simulink model "HSat_orbit_merged_maria"  (R2023b)
settings: Solver=FixedStepAuto  StartTime=0  StopTime=86400*900  MaxStep=3600  RelTol=1e-3  EnableMultiTasking=on
values from neighbouring files (symbols this model uses):
  alpha_acc = sqrt(0.7)    [HSat_op_setup_merged_maria.m]    (also in init_orbit_analysis_with_drag_loss.m)
  ext_ENV_G = 6.674e-11    [HSat_op_setup.m]    (also in HSat_op_setup_merged_maria.m)
  ext_ENV_muEarth = 3.986005e14    (= 398600500000000)    [GEO_insertion_setup.m]    (also in HSat_op_setup.m; HSat_op_setup_merged_maria.m; init_orbit_analysis_with_drag_loss.m)
  ext_ENV_Re = 6.37813700*10^6    (= 6378137)    [HSat_op_setup.m]    (also in HSat_op_setup_merged_maria.m)
  ext_EOR_atmosphere_end = 1000e3    (= 1000000)    [HSat_op_setup.m]    (also in HSat_op_setup_merged_maria.m)
  ext_EOR_perigeeraise_end = 600e3    (= 600000)    [HSat_op_setup.m]    (also in HSat_op_setup_merged_maria.m)
  ext_Main_initDate_IC_T = sim_start    [HSat_op_setup.m]    (also in HSat_op_setup_merged_maria.m)
  ext_SC_activecorr_COE_ECI = [1, 1, 1, 0, 0, 0, 0, 0 ]    [HSat_op_setup.m]    (also in HSat_op_setup_merged_maria.m)
  ext_SC_balanced_COE_ECI = [ .500    0.70    1.100 1 1]    [HSat_op_setup.m]    (also in HSat_op_setup_merged_maria.m = [ 0.10 2.10 1.40    1.0000    1.0000]; launch_settings.m)
  ext_SC_cutofferror_COE_ECI = [150e3, .01, 0.1*pi/180, .1*pi/180,.1*pi/180, 0, 0, 0]    [HSat_op_setup.m]    (also in HSat_op_setup_merged_maria.m)
  ext_SC_init_COE_ECI = [a0,ecc0,i0,an0,ap0,tran0,eccan0,ma0]    [HSat_op_setup.m]    (also in HSat_op_setup_merged_maria.m)
  ext_SC_target_COE_ECI = [a1,ecc1,i1,an1,ap1,tran1,eccan1,ma1]    [HSat_op_setup.m]    (also in HSat_op_setup_merged_maria.m)
  ext_SC_target_lambda = 67*pi/180    (= 1.16937059884)    [HSat_op_setup.m]    (also in HSat_op_setup_merged_maria.m)
  flip_timer = 2*60*60    (= 7200)    [HSat_op_setup_merged_maria.m]
  P_solar = 4.56e-6    (= 4.56e-06)    [HSat_op_setup_merged_maria.m]    (also in init_orbit_analysis_with_drag_loss.m)
  sim_SC_init_CoG_EOR_dry = [-0.00448 0.00106 0.46931]    [HSat_op_setup.m]    (also in HSat_op_setup_merged_maria.m)
  sim_SC_init_CoG_propellant = [0 0 0.24758]    [HSat_op_setup.m]    (also in HSat_op_setup_merged_maria.m)
  sim_SC_init_dry_mass = sim_SC_init_wet_mass-sim_SC_init_propellant_mass    (= 727)    [HSat_op_setup.m]    (also in HSat_op_setup_merged_maria.m = 813.7)
  sim_SC_init_MoI_EOR_wet = [ ... (first row only)    [HSat_op_setup.m]    (also in HSat_op_setup_merged_maria.m; init_orbit_analysis_with_drag_loss.m)
  sim_SC_init_wet_mass = 750    [HSat_op_setup.m]    (also in HSat_op_setup_merged_maria.m)
  sim_thrust_force = [ ... (first row only)    [HSat_op_setup.m]    (also in HSat_op_setup_merged_maria.m)
  sim_thrust_massflow = [ ... (first row only)    [HSat_op_setup.m]    (also in HSat_op_setup_merged_maria.m)
  sim_thrust_vector = [ ... (first row only)    [HSat_op_setup.m]    (also in HSat_op_setup_merged_maria.m)
  sim_thruster_position = [ ... (first row only)    [HSat_op_setup.m]    (also in HSat_op_setup_merged_maria.m)
  sim_ts_save = 60    [HSat_op_setup.m]    (also in HSat_op_setup_merged_maria.m)
  sun_pointing_SA = 0    [HSat_op_setup_merged_maria.m]    (also in init_orbit_analysis_with_drag_loss.m)
  third_body_jupiter = 1    [HSat_op_setup.m]    (also in HSat_op_setup_merged_maria.m)
  third_body_moon = 1    [HSat_op_setup.m]    (also in HSat_op_setup_merged_maria.m)
  third_body_sun = 1    [HSat_op_setup.m]    (also in HSat_op_setup_merged_maria.m)
libraries: aerolibutil x59, simulink x18, matrix_library x16, Toolbox x10, sharedtransform x9, sharedutil x5, aerolibatmos2 x1, simulink_extras x1
(part 2 of 8)

== system HSat_orbit_merged_maria/Subsystem1/Navigation/q_slo ==
  posECI : Inport
  velECI : Inport  Port=2
  Create 3x3 Matrix : sharedutil/Create 3x3 Matrix  aMode=aMode
      settings: LibrarySourceBlock=aerolibutil/Create 3x3 Matrix
  Demux : Demux  Outputs=3
  Demux1 : Demux  Outputs=3
  Demux2 : Demux  Outputs=3
  Direction Cosine Matrix to Quaternions : sharedtransform/Direction Cosine Matrix  to Quaternions  aMode=0  action=None  tolerance=eps(2)
      settings: LibrarySourceBlock=|
      | aerolibtransform2/Direction Cosine Matrix
      | to Quaternions
  Unary Minus : UnaryMinus
  VecNormalize : Subsystem
      mask Display: disp('u/||u||')
  VecNormalize1 : Subsystem
      mask Display: disp('u/||u||')
  VecNormalize2 : Subsystem
      mask Display: disp('u/||u||')
  VecNormalize3 : Subsystem
      mask Display: disp('u/||u||')
  Z x R : Subsystem  mask(Cross Product){}
      mask help: Calculates the cross product of two 3x1 vectors.
      mask Help:
      | <p>This block calculates the cross product of two 3x1 vectors, ie.</p>
      | 
      | <ul>C(1) = A(2)*B(3) - A(3)*B(2)</ul>
      | <ul>C(2) = A(3)*B(1) - A(1)*B(3)</ul>
      | <ul>C(3) = A(1)*B(2) - A(2)*B(1)</ul>
      | 
      | <p>The block inputs and output contain more than one signal as described below.</p>
      | 
      | <p><H4>Block Vector Input 1 - A</H4>
      | <ul>
      | <li>A(1)</li>
      | <li>A(2)</li>
      | <li>A(3)</li>
      | </ul>
      | </p>
      | 
      | <p><H4>Block Vector Input 2 - B</H4>
      | <ul>
      | <li>B(1)</li>
      | <li>B(2)</li>
      | <li>B(3)</li>
      | </ul>
      | </p>
      | 
      | <p><H4>Block Vector Output - Cross Product (AxB)</H4>
      | <ul>
      | <li>C(1)</li>
      | <li>C(2)</li>
      | <li>C(3)</li>
      | </ul>
      | </p>
      mask Display: disp('Cross\nProduct')
  Z x Y : Subsystem  mask(Cross Product){}
      mask help: Calculates the cross product of two 3x1 vectors.
      mask Help:
      | <p>This block calculates the cross product of two 3x1 vectors, ie.</p>
      | 
      | <ul>C(1) = A(2)*B(3) - A(3)*B(2)</ul>
      | <ul>C(2) = A(3)*B(1) - A(1)*B(3)</ul>
      | <ul>C(3) = A(1)*B(2) - A(2)*B(1)</ul>
      | 
      | <p>The block inputs and output contain more than one signal as described below.</p>
      | 
      | <p><H4>Block Vector Input 1 - A</H4>
      | <ul>
      | <li>A(1)</li>
      | <li>A(2)</li>
      | <li>A(3)</li>
      | </ul>
      | </p>
      | 
      | <p><H4>Block Vector Input 2 - B</H4>
      | <ul>
      | <li>B(1)</li>
      | <li>B(2)</li>
      | <li>B(3)</li>
      | </ul>
      | </p>
      | 
      | <p><H4>Block Vector Output - Cross Product (AxB)</H4>
      | <ul>
      | <li>C(1)</li>
      | <li>C(2)</li>
      | <li>C(3)</li>
      | </ul>
      | </p>
      mask Display: disp('Cross\nProduct')
  qECI2slo : Outport  InitialOutput=0
  wires:
  Unary Minus/1 -> Z x Y/2(b(1) b(2) b(3)), Demux2/1, Z x R/1(a(1) a(2) a(3))  "Z"
  posECI/1 -> VecNormalize3/1(In1)
  VecNormalize3/1(Out1) -> Unary Minus/1
  velECI/1 -> VecNormalize2/1(In1)
  VecNormalize2/1(Out1) -> Z x R/2(b(1) b(2) b(3))
  Z x R/1(c(1) c(2) c(3)) -> VecNormalize1/1(In1)
  VecNormalize1/1(Out1) -> Z x Y/1(a(1) a(2) a(3)), Demux1/1  "Y"
  Z x Y/1(c(1) c(2) c(3)) -> VecNormalize/1(In1)
  VecNormalize/1(Out1) -> Demux/1  "X"
  Demux/1 -> Create 3x3 Matrix/1
  Demux/2 -> Create 3x3 Matrix/2
  Demux/3 -> Create 3x3 Matrix/3
  Demux1/1 -> Create 3x3 Matrix/4
  Demux1/2 -> Create 3x3 Matrix/5
  Demux1/3 -> Create 3x3 Matrix/6
  Demux2/1 -> Create 3x3 Matrix/7
  Demux2/2 -> Create 3x3 Matrix/8
  Demux2/3 -> Create 3x3 Matrix/9
  Create 3x3 Matrix/1 -> Direction Cosine Matrix to Quaternions/1
  Direction Cosine Matrix to Quaternions/1 -> qECI2slo/1

== system HSat_orbit_merged_maria/Subsystem1/control/EORattitude ==
  note: Not used
  AllThrustsSCB : Inport
  AmomECI : Inport  Port=2
  thrust_slo : Inport  Port=3
  sunv_eci : Inport  Port=4
  q_eci2slo : Inport  Port=5
  AllTorquesSCB1 : Inport  Port=6
  q_eci2scb : Inport  Port=7
  Bus Creator : BusCreator  Inputs=3
  Bus Creator1 : BusCreator  Inputs=3
  Bus Selector : BusSelector  OutputSignals=signal1,signal2,signal3
  Delay : Delay  DelayLength=1  InitialCondition=0
  Logical Operator : Logic  Operator=OR  AllPortsSameDT=off  OutDataTypeStr=boolean
  Logical Operator1 : Logic  Operator=NOT  AllPortsSameDT=off  OutDataTypeStr=boolean
  Logical Operator2 : Logic  AllPortsSameDT=off  OutDataTypeStr=boolean
  Manual Switch1 : ManualSwitch  CurrentSetting=0
  OR or SK unloading : Subsystem
  Subsystem : Subsystem
  Subsystem2 : Subsystem
  Subsystem4 : Subsystem
  Terminator : Terminator
  Unit Delay : UnitDelay  SampleTime=-1  HasFrameUpgradeWarning=on
  ActiveThrusters : Outport
  qECI2scb : Outport  Port=2
  DoAMOM : Outport  Port=3
  flip_unload : Outport  Port=4
  wires:
  sunv_eci/1 -> Subsystem/7(sunv_eci), Subsystem4/6(sunv_eci)
  Subsystem2/3(EORTorqueSCB) -> Subsystem4/3(EORtorqueSCB), Subsystem/4(EORtorqueSCB)
  AmomECI/1 -> OR or SK unloading/1(AmomECI), Subsystem4/1(AmomECI), Subsystem/1(AmomECI)
  Subsystem4/1(qECI2scb) -> Bus Creator1/1
  Subsystem2/2(EORForceSCB) -> Subsystem4/2(EORthrustSCB), Subsystem/3(EORthrustSCB)
  thrust_slo/1 -> Subsystem4/4(thrust_slo), Subsystem/5(thrust_slo)
  q_eci2slo/1 -> Subsystem4/5(q_eci2slo), Subsystem/6(q_slo2eci)
  Subsystem/1(qECI2scb) -> Bus Creator/1
  OR or SK unloading/1(PPU1active) -> Subsystem2/1(PPU1active)
  AllThrustsSCB/1 -> Subsystem2/2(AllThrustsSCB)
  OR or SK unloading/2(PPU2active) -> Subsystem2/3(PPU2active)
  AllTorquesSCB1/1 -> Subsystem2/4(AllTorquesSCB1)
  Subsystem2/1(ActiveThrusters) -> ActiveThrusters/1
  q_eci2scb/1 -> Subsystem/2(q_eci2scb)
  Subsystem4/2(DoAMOM) -> Bus Creator1/2
  Subsystem/2(DoAMOM) -> Bus Creator/2
  Bus Creator1/1 -> Manual Switch1/2
  Bus Creator/1 -> Manual Switch1/1
  Manual Switch1/1 -> Bus Selector/1
  Bus Selector/1 -> qECI2scb/1  "<signal1>"
  Bus Selector/2 -> Logical Operator/1  "<signal2>"
  Subsystem4/3(NoAMOM) -> Bus Creator1/3
  Subsystem/3(NoAMOM) -> Bus Creator/3
  Bus Selector/3 -> Logical Operator1/1  "<signal3>"
  Logical Operator1/1 -> Logical Operator2/2
  Logical Operator2/1 -> DoAMOM/1, Delay/1
  Delay/1 -> Logical Operator/2
  Logical Operator/1 -> Logical Operator2/1
  OR or SK unloading/3(PPUSKactive) -> Subsystem4/7(unloading_ongoing), Subsystem2/5(PPUSKactive)
  Subsystem2/4(SKThrustersActive) -> Terminator/1
  Subsystem4/5(SKunload) -> Unit Delay/1
  Unit Delay/1 -> OR or SK unloading/2(SKunload)
  Subsystem4/4(flip_unloading) -> flip_unload/1

== system HSat_orbit_merged_maria/Subsystem1/control/Subsystem6 ==
  q_eci2scb_wanted : Inport
  AllTorquesSCB : Inport  Port=2
  sunv : Inport  Port=3
  WantedTorqueECI : Inport  Port=4
  PPU1active : Inport  Port=5
  PPU2active : Inport  Port=6
  Subsystem2 : Subsystem
  active_thrusters : Outport
  q_eci2scb : Outport  Port=2
  wires:
  AllTorquesSCB/1 -> Subsystem2/3(AllTorquesSCB)
  q_eci2scb_wanted/1 -> Subsystem2/4(q_eci2scb_wanted)
  PPU1active/1 -> Subsystem2/1(PPU1active)
  PPU2active/1 -> Subsystem2/2(PPU2active)
  WantedTorqueECI/1 -> Subsystem2/5(WantedTorqueECI)
  Subsystem2/1(ActiveThrusters) -> active_thrusters/1
  Subsystem2/2(q_eci2scb) -> q_eci2scb/1
  sunv/1 -> Subsystem2/6(sunv)

== system HSat_orbit_merged_maria/Subsystem1/control/TorquesAndForces ==
  Active_thruster : Inport
  thrusting : Inport  Port=2
  SC_mass : Inport  Port=3
  Constant : Constant  Value=sim_thruster_position
  Constant1 : Constant  Value=sim_thrust_vector
  Constant2 : Constant  Value=sim_thrust_force
  Constant3 : Constant  Value=[1 1 1]
  Constant4 : Constant  Value=[1 1 1 1 1 1 1 1 1 1 1]'
  Constant5 : Constant  Value=sim_thrust_massflow
  Constant6 : Constant  Value=[1 1 1]
  Display : Display
  MATLAB Function : MATLAB Function  TreatAsAtomicUnit=on
  Product{,2,4..5,7} (5 alike) : Product
  Product1 : Product  Multiplication=Matrix(*)
  Product3 : Product  Multiplication=Matrix(*)
  Product6 : Product  Multiplication=Matrix(*)
  Reshape : Reshape  OutputDimensionality=Column vector (2-D)
  Reshape1 : Reshape  OutputDimensionality=Column vector (2-D)
  Reshape2 : Reshape  OutputDimensionality=Row vector (2-D)
  Reshape3 : Reshape  OutputDimensionality=Row vector (2-D)
  Reshape4 : Reshape  OutputDimensionality=Column vector (2-D)
  Subsystem : Subsystem
  Sum : Sum  Inputs=+-|
  Sum of Elements1 : Sum  Inputs=+  CollapseMode=Specified dimension
  Sum of Elements2 : Sum  Inputs=+  CollapseMode=Specified dimension
  Sum of Elements6 : Sum  Inputs=+  CollapseMode=Specified dimension
  EPtorqueSCB : Outport
  EPThrustSCB : Outport  Port=2
  TotalMassFlow : Outport  Port=3
  AllThrustsSCB : Outport  Port=4
  AllTorquesSCB : Outport  Port=5
  wires:
  Sum of Elements6/1 -> EPtorqueSCB/1
  Sum of Elements1/1 -> EPThrustSCB/1
  Product5/1 -> Sum of Elements6/1
  SC_mass/1 -> Subsystem/1(SC_mass)
  Constant2/1 -> Reshape1/1
  Sum/1 -> MATLAB Function/1(v)
  Subsystem/1(SC_CoG) -> Product3/2
  Reshape1/1 -> Product1/1
  Constant1/1 -> Product2/1
  Product1/1 -> Product2/2
  Constant/1 -> Sum/1
  Constant4/1 -> Product3/1
  Constant3/1 -> Reshape2/1
  Reshape2/1 -> Product1/2
  Product3/1 -> Sum/2
  Reshape4/1 -> Product4/1
  Constant5/1 -> Reshape4/1
  Product4/1 -> Sum of Elements2/1
  Sum of Elements2/1 -> TotalMassFlow/1
  Product/1 -> Sum of Elements1/1
  MATLAB Function/1(u) -> AllTorquesSCB/1, Product5/1
  Product6/1 -> Product5/2, Product/2
  Constant6/1 -> Reshape3/1
  Reshape3/1 -> Product6/2
  Reshape/1 -> Product4/2, Product6/1
  thrusting/1 -> Product7/2
  Product7/1 -> Reshape/1
  Product2/1 -> Product/1, AllThrustsSCB/1, MATLAB Function/2(w)
  Active_thruster/1 -> Display/1, Product7/1

== system HSat_orbit_merged_maria/Subsystem1/Dynamics/Subsystem/3 body perturbation legendre polynomial ==
  r_sat : Inport
  r_sun : Inport  Port=2
  r_moon : Inport  Port=3
  r_jupiter : Inport  Port=4
  Constant1 : Constant  Value=[0,0,0]
  Constant2 : Constant  Value=[0,0,0]
  Constant3 : Constant  Value=third_body_sun
  Constant4 : Constant  Value=third_body_moon
  Constant5 : Constant  Value=[0,0,0]
  Constant6 : Constant  Value=third_body_jupiter
  Legendre degree : Constant  Value=2
  Subsystem1 : Subsystem
  Subsystem2 : Subsystem
  Subsystem3 : Subsystem
  Subtract : Sum  Inputs=---
  Switch1 : Switch  Criteria=u2 > Threshold  SaturateOnIntegerOverflow=off  InputSameDT=off
  Switch2 : Switch  Criteria=u2 > Threshold  SaturateOnIntegerOverflow=off  InputSameDT=off
  Switch3 : Switch  Criteria=u2 > Threshold  SaturateOnIntegerOverflow=off  InputSameDT=off
  jupiter mass : Constant  Value=1.898e27
  moon mass : Constant  Value=7.342e22
  sun mass : Constant  Value=1.989e30
  3rdbodyacc : Outport
  wires:
  r_sat/1 -> Subsystem1/1(sat), Subsystem3/1(sat), Subsystem2/1(sat)
  r_sun/1 -> Subsystem2/2(3 body)
  sun mass/1 -> Subsystem2/3(mass)
  r_moon/1 -> Subsystem1/2(3 body)
  moon mass/1 -> Subsystem1/3(mass)
  r_jupiter/1 -> Subsystem3/2(3 body)
  jupiter mass/1 -> Subsystem3/3(mass)
  Subtract/1 -> 3rdbodyacc/1
  Legendre degree/1 -> Subsystem1/4(Legendre deg), Subsystem3/4(Legendre deg), Subsystem2/4(Legendre deg)
  Subsystem2/1(Out1) -> Switch1/1
  Switch1/1 -> Subtract/1
  Constant2/1 -> Switch1/3
  Constant3/1 -> Switch1/2
  Constant1/1 -> Switch2/3
  Switch2/1 -> Subtract/2
  Constant4/1 -> Switch2/2
  Subsystem1/1(Out1) -> Switch2/1
  Constant5/1 -> Switch3/3
  Switch3/1 -> Subtract/3
  Constant6/1 -> Switch3/2
  Subsystem3/1(Out1) -> Switch3/1

== system HSat_orbit_merged_maria/Subsystem1/Dynamics/Subsystem/Ephemeris ==
  T JD : Inport
  Gain{,1..3} (4 alike) : Gain  Gain=1000
  Jupiter Ephemeris : PlanetaryEphem  target=Jupiter
  Lunar Ephemeris : PlanetaryEphem
  Solar Ephemeris : PlanetaryEphem  target=Sun
  Terminator : Terminator
  Terminator1 : Terminator
  Terminator2 : Terminator
  km to m : Gain  Gain=1000
  km to m1 : Gain  Gain=1000
  solar_X : Outport
  lunar_X : Outport  Port=2
  jupiter_X : Outport  Port=3
  wires:
  T JD/1 -> Lunar Ephemeris/1, Jupiter Ephemeris/1, Solar Ephemeris/1
  Lunar Ephemeris/2 -> Gain1/1
  Solar Ephemeris/1 -> Gain2/1
  Solar Ephemeris/2 -> km to m/1
  Lunar Ephemeris/1 -> Gain/1
  Gain/1 -> lunar_X/1
  Gain1/1 -> Terminator2/1
  Gain2/1 -> solar_X/1
  km to m/1 -> Terminator1/1
  Jupiter Ephemeris/2 -> km to m1/1
  Gain3/1 -> jupiter_X/1
  km to m1/1 -> Terminator/1
  Jupiter Ephemeris/1 -> Gain3/1

== system HSat_orbit_merged_maria/Subsystem1/Dynamics/disturbing torques/Atmospheric model ==
  pos_ECI : Inport
  julianDate : Inport  Port=2
  qECI2ECEF : Inport  Port=3
  F107 : Constant  Value=150
  F107a : Constant  Value=150
  MATLAB Function1 : MATLAB Function  TreatAsAtomicUnit=on
  NRLMSISE-00 Atmosphere Model : aerolibatmos2/NRLMSISE-00 Atmosphere Model  units=Metric (MKS)  lst_input=off  flux_ap_input=on  flags_input=Internal  flags=ones(1,23)  oxygen_in=off  action=Warning
  aph : Constant  Value=17*ones(1,7)
  pos_eci to lla : Subsystem
  T : Outport
  rho : Outport  Port=2
  wires:
  NRLMSISE-00 Atmosphere Model/2 -> rho/1
  qECI2ECEF/1 -> pos_eci to lla/2(qECI2ECEF)
  julianDate/1 -> MATLAB Function1/1(julianDate)
  F107/1 -> NRLMSISE-00 Atmosphere Model/6
  NRLMSISE-00 Atmosphere Model/1 -> T/1
  MATLAB Function1/1(yr) -> NRLMSISE-00 Atmosphere Model/2
  pos_ECI/1 -> pos_eci to lla/1(pos_ECI)
  aph/1 -> NRLMSISE-00 Atmosphere Model/7
  MATLAB Function1/2(dayOfYear) -> NRLMSISE-00 Atmosphere Model/3
  pos_eci to lla/1(Out1) -> NRLMSISE-00 Atmosphere Model/1  "lat,long,alt"
  F107a/1 -> NRLMSISE-00 Atmosphere Model/5
  MATLAB Function1/3(timeUTSeconds) -> NRLMSISE-00 Atmosphere Model/4

== system HSat_orbit_merged_maria/Subsystem1/Dynamics/disturbing torques/Disturbing torques ==
  SC_CoG : Inport
  qECI2scb : Inport  Port=2
  vel_eci : Inport  Port=3
  pos_eci : Inport  Port=4
  rho : Inport  Port=5
  solar_X : Inport  Port=6
  ECI to SCB : Subsystem
  Gravity gradient torque : Subsystem
  Total ang_mom ECI : Sum  Inputs=+++
  Total torque ECI : Sum  Inputs=+++
  sc area projected to v / aero drag torque / srp torque : Subsystem
      settings: PortSchema="{\"entries\":[{\"content\":{\"sides\":[{\"content\":{\"connectorIds\":[\"Out5\",\"Out6\",\"Out7\"]},\"type\":\"ConnectorPlacement.EquallySpacedRectSide\",\"uuid\":\"2286bbd5-74fd-4e7a-af53-1dba63e33399\"},{\"content\":{\"connectorIds\":[\"Out1\",\"Out2\",\"Out3\",\"Out4\"],\"side\":\"RIGHT\"},\"type\":\"ConnectorPlacement.EquallySpacedRectSide\",\"uuid\":\"14ee861f-d330-4e3d-9d37-eadf89803ba2\"},{\"content\":{\"connectorIds\":[\"In1\",\"In2\",\"In3\",\"In4\",\"In5\",\"In6\"],\"side\":\"TOP\"},\"type\":\"ConnectorPlacement.EquallySpacedRectSide\",\"uuid\":\"a82f7821-7262-41d9-9ef8-416bfb7d6f77\"}]},\"type\":\"ConnectorPlacement.EquallySpacedConnector\",\"uuid\":\"26570817-76bd-4bb8-9b49-7b0dee7f17a2\"}],\"packageUris\":[\"http://schema.mathworks.com/mf0/Connector/R2020b\"],\"version\":\"1.0\"}"
  N_gg_scb : Outport
  L_gg_scb : Outport  Port=2
  L_aero_scb : Outport  Port=3
  L_srp_scb : Outport  Port=4
  N_gg_eci : Outport  Port=5
  N_total_scb : Outport  Port=6
  L_gg_eci : Outport  Port=7
  L_total_scb : Outport  Port=8
  N_total_ECI : Outport  Port=9
  L_total_ECI : Outport  Port=10
  N_aero_eci : Outport  Port=11
  L_aero_eci : Outport  Port=12
  N_aero_scb : Outport  Port=13
  N_srp_eci : Outport  Port=14
  L_srp_eci : Outport  Port=15
  N_srp_scb : Outport  Port=16
  proj_area : Outport  Port=17
  wires:
  pos_eci/1 -> Gravity gradient torque/2(pos), sc area projected to v / aero drag torque / srp torque/4(pos_eci)
  sc area projected to v / aero drag torque / srp torque/5(proj_area) -> proj_area/1
  Gravity gradient torque/2(L_gg_eci) -> L_gg_eci/1, Total ang_mom ECI/1, ECI to SCB/3(L_gg_eci)
  sc area projected to v / aero drag torque / srp torque/4(L_srp_eci) -> ECI to SCB/5(L_srp_eci), Total ang_mom ECI/3, L_srp_eci/1
  rho/1 -> sc area projected to v / aero drag torque / srp torque/2(rho)
  ECI to SCB/4(L_srp_scb) -> L_srp_scb/1
  ECI to SCB/5(N_total_scb) -> N_total_scb/1
  solar_X/1 -> sc area projected to v / aero drag torque / srp torque/6(solar_X)
  ECI to SCB/3(L_aero_scb) -> L_aero_scb/1
  sc area projected to v / aero drag torque / srp torque/3(N_srp_eci) -> Total torque ECI/3, N_srp_eci/1
  Total torque ECI/1 -> ECI to SCB/6(N_total_ECI), N_total_ECI/1
  ECI to SCB/6(L_total_scb) -> L_total_scb/1
  ECI to SCB/2(L_gg_scb) -> L_gg_scb/1
  sc area projected to v / aero drag torque / srp torque/1(N_aero_eci) -> Total torque ECI/2, N_aero_eci/1
  ECI to SCB/1(N_gg_scb) -> N_gg_scb/1
  Total ang_mom ECI/1 -> ECI to SCB/7(L_total_ECI), L_total_ECI/1
  qECI2scb/1 -> ECI to SCB/1(qECI2scb), sc area projected to v / aero drag torque / srp torque/3(qECI2scb), Gravity gradient torque/1(qECI2scb)
  sc area projected to v / aero drag torque / srp torque/7(N_srp_scb) -> N_srp_scb/1
  Gravity gradient torque/1(N_gg_eci) -> Total torque ECI/1, N_gg_eci/1, ECI to SCB/2(N_gg_eci)
  sc area projected to v / aero drag torque / srp torque/6(N_aero_scb) -> N_aero_scb/1
  vel_eci/1 -> sc area projected to v / aero drag torque / srp torque/5(vel_eci)
  sc area projected to v / aero drag torque / srp torque/2(L_aero_eci) -> ECI to SCB/4(L_aero_eci), Total ang_mom ECI/2, L_aero_eci/1
  SC_CoG/1 -> sc area projected to v / aero drag torque / srp torque/1(SC_CoG)

== system HSat_orbit_merged_maria/Subsystem1/Dynamics/disturbing torques/Subsystem ==
  SC_mass : Inport
  Constant1 : Constant  Value=sim_SC_init_CoG_EOR_dry
  Constant2 : Constant  Value=sim_SC_init_CoG_propellant
  Constant3 : Constant  Value=sim_SC_init_dry_mass
  Constant4 : Constant  Value=sim_SC_init_dry_mass
  Divide : Product  Inputs=/*
  Product : Product
  Product1 : Product
  Reshape : Reshape  OutputDimensionality=Row vector (2-D)
  Sum : Sum  Inputs=+-|
  Sum1 : Sum  Inputs=+|+
  SC_CoG : Outport
  wires:
  Constant4/1 -> Sum/2
  Product1/1 -> Sum1/2
  Constant3/1 -> Product1/1
  SC_mass/1 -> Divide/1, Sum/1
  Constant1/1 -> Product1/2
  Product/1 -> Sum1/1
  Sum1/1 -> Divide/2
  Constant2/1 -> Product/2
  Sum/1 -> Product/1  "propellant mass"
  Divide/1 -> Reshape/1
  Reshape/1 -> SC_CoG/1

== system HSat_orbit_merged_maria/Subsystem1/Guidance/Subsystem1/Subsystem ==
  coe : Inport
  activecorr : Inport  Port=2
  coe1 : Inport  Port=3
  symelems : Inport  Port=4
  lambda1 : Inport  Port=5
  Abs : Abs  SaturateOnIntegerOverflow=off
  Bus Selector1 : BusSelector  OutputSignals=lambdadot,lambdaM
  Bus Selector2 : BusSelector  OutputSignals=sms
  Compare To Constant : simulink/Logic and Bit Operations/Compare To Constant  relop=<=  const=4  OutDataTypeStr=boolean
  Gain : Gain  Gain=180/pi
  Gain1 : Gain  Gain=180/pi
  Gain2 : Gain  Gain=180/pi
  Gain3 : Gain  Gain=.5
  Mux : Mux  Inputs=2
  Scope1 : Scope  NumInputPorts=3
  Scope2 : Scope  NumInputPorts=2
  Selector : Selector  InputPortWidth=8  IndexOptions=Index vector (dialog)  Indices=[2 3 4 5 6 7 8]  OutputSizes=1
  Subsystem1 : Subsystem
  Sum : Sum  Inputs=-+|
  plusminuspi : Subsystem
  NEARGEO : Outport
  ACTIVECORR : Outport  Port=2
  COE1 : Outport  Port=3
  wires:
  coe1/1 -> Selector/1
  coe/1 -> Bus Selector2/1
  lambda1/1 -> Sum/2
  symelems/1 -> Bus Selector1/1
  Abs/1 -> Compare To Constant/1
  Gain3/1 -> Gain1/1, Subsystem1/1(lambdadot_guide)
  Sum/1 -> plusminuspi/1(lambda)
  Selector/1 -> Mux/2
  Gain1/1 -> Scope1/2
  Gain2/1 -> Scope1/1
  Bus Selector1/1 -> Gain/1  "<lambdadot>"
  Bus Selector1/2 -> Sum/1  "<lambdaM>"
  Subsystem1/1(a_guide) -> Scope2/1, Mux/1
  Bus Selector2/1 -> Scope2/2  "<sms>"
  plusminuspi/1(lambdadot_guide) -> Gain2/1, Gain3/1
  Mux/1 -> COE1/1
  Gain/1 -> Scope1/3, Abs/1
  Compare To Constant/1 -> NEARGEO/1
  activecorr/1 -> ACTIVECORR/1

== system HSat_orbit_merged_maria/Subsystem1/Guidance/Subsystem1/perigeerraise ==
  coe : Inport
  "activecorr_coe " : Inport  Port=2
  Coe1 : Inport  Port=3
  Bus Selector : BusSelector  OutputSignals=sms
  Compare To Constant : simulink/Logic and Bit Operations/Compare To Constant  relop=<=  const=ext_EOR_perigeeraise_end  OutDataTypeStr=boolean
  Gain4 : Gain  Gain=[1 0 0 0 0 0 0 0]
  Gain5 : Gain  Gain=1.1
  Mux1 : Mux  Inputs=2
  Selector2 : Selector  InputPortWidth=8  IndexOptions=Index vector (dialog)  Indices=[2 3 4 5 6 7 8]  OutputSizes=1
  Subsystem2 : Subsystem
  Terminator : Terminator
  PERIGEEISLOW : Outport
  ACTIVECORR : Outport  Port=2
  COE1 : Outport  Port=3
  wires:
  Coe1/1 -> Selector2/1
  Compare To Constant/1 -> PERIGEEISLOW/1
  Subsystem2/2(Apogee altitude) -> Terminator/1
  "activecorr_coe "/1 -> Gain4/1
  Selector2/1 -> Mux1/2
  Subsystem2/1(Perigee altitude) -> Compare To Constant/1
  coe/1 -> Bus Selector/1, Subsystem2/1(COE)
  Gain4/1 -> ACTIVECORR/1
  Mux1/1 -> COE1/1
  Bus Selector/1 -> Gain5/1  "<sms>"
  Gain5/1 -> Mux1/1

== system HSat_orbit_merged_maria/Subsystem1/Navigation/Subsystem/Subsystem ==
  posECI : Inport
  velECI : Inport  Port=2
  Bus Creator : BusCreator  Inputs=11
  Demux : Demux  Outputs=11
  MATLAB Function : MATLAB Function  TreatAsAtomicUnit=on
  coe : Outport
  wires:
  posECI/1 -> MATLAB Function/1(r)
  Demux/10 -> Bus Creator/10  "truelong"
  Demux/1 -> Bus Creator/1  "sms"
  Demux/3 -> Bus Creator/3  "incl"
  Demux/7 -> Bus Creator/7  "eccan"
  Demux/9 -> Bus Creator/9  "arglat"
  Demux/4 -> Bus Creator/4  "raan"
  Demux/2 -> Bus Creator/2  "ecc"
  Demux/11 -> Bus Creator/11  "longper"
  Demux/6 -> Bus Creator/6  "truean"
  MATLAB Function/1(coe) -> Demux/1
  Bus Creator/1 -> coe/1  "coe"
  velECI/1 -> MATLAB Function/2(v)
  Demux/5 -> Bus Creator/5  "argp"
  Demux/8 -> Bus Creator/8  "meanan"

== system HSat_orbit_merged_maria/Subsystem1/Navigation/Subsystem/Subsystem2 ==
  jd : Inport
  epoch_jd : Inport  Port=2
  pos_ECI : Inport  Port=3
  vel_ECI : Inport  Port=4
  Bus Creator : BusCreator  Inputs=12
  Bus Creator1 : BusCreator  Inputs=10
  Bus Selector : BusSelector  OutputSignals=jd,epoch_jd,Raan,argp,nu,a,M,e,h
  Subsystem1 : Subsystem
  Subsystem7 : Subsystem
  Terminator : Terminator
  SyncElems : Outport
  wires:
  pos_ECI/1 -> Subsystem7/1(r)  "r"
  vel_ECI/1 -> Subsystem7/2(v)  "v"
  Subsystem7/9(e) -> Bus Creator/9
  Subsystem7/2(eabs) -> Bus Creator/2
  Subsystem7/10(h) -> Bus Creator/10
  Subsystem7/3(i) -> Bus Creator/3
  Subsystem7/5(argp) -> Bus Creator/5
  Subsystem7/4(Raan) -> Bus Creator/4
  Subsystem7/1(a) -> Bus Creator/1
  Subsystem7/6(nu) -> Bus Creator/6
  jd/1 -> Bus Creator/11  "jd"
  Bus Creator/1 -> Bus Selector/1
  Bus Selector/4 -> Subsystem1/4(<argp>)  "<argp>"
  Bus Selector/1 -> Subsystem1/1(<jd>)  "<jd>"
  Bus Selector/5 -> Subsystem1/5(<nu>)  "<nu>"
  Bus Selector/3 -> Subsystem1/3(<Raan>)  "<Raan>"
  Subsystem7/8(M) -> Bus Creator/8
  Subsystem7/7(E) -> Bus Creator/7
  Subsystem7/11(nu igen) -> Terminator/1
  epoch_jd/1 -> Bus Creator/12  "epoch_jd"
  Bus Selector/2 -> Subsystem1/2(epoch_jd)  "<epoch_jd>"
  Bus Selector/7 -> Subsystem1/7(M)  "<M>"
  Bus Selector/6 -> Subsystem1/6(a)  "<a>"
  Bus Selector/8 -> Subsystem1/8(e)  "<e>"
  Bus Selector/9 -> Subsystem1/9(h)  "<h>"
  Subsystem1/1(jd) -> Bus Creator1/1  "jd"
  Subsystem1/2(epochJd) -> Bus Creator1/2  "epochjd"
  Subsystem1/3(lambda) -> Bus Creator1/3  "lambda"
  Subsystem1/4(lambdaM) -> Bus Creator1/4  "lambdaM"
  Subsystem1/5(lambda0) -> Bus Creator1/5  "lambda0"
  Subsystem1/6(lambda_dot) -> Bus Creator1/6  "lambdadot"
  Subsystem1/7(ex) -> Bus Creator1/7  "ex"
  Subsystem1/9(ix) -> Bus Creator1/9  "ix"
  Bus Creator1/1 -> SyncElems/1
  Subsystem1/8(ey) -> Bus Creator1/8  "ey"
  Subsystem1/10(iy) -> Bus Creator1/10  "iy"

== system HSat_orbit_merged_maria/Subsystem1/Navigation/Subsystem8/Simplified Shadow Fraction ==
  note: Compute angular radius rho of Earth as viewed from ISS
  note: If dot product of normalized satellite position vector and sun vectors is smaller than cos rho then Earth is not blocking sun.
  x_sun_icrf : Inport  SampleTime=0
  X_icrf : Inport  Port=2
  Acos : Trigonometry  Operator=asin
  Acos1 : Trigonometry  Operator=cos
  Constant : Constant  Value=eps
  Constant1 : Constant  Value=eps
  Divide : Product  Inputs=/*
  Divide1 : Product  Inputs=*/
  Divide2 : Product  Inputs=/*
  Dot Product1 : DotProduct  OutDataTypeStr=Inherit: Inherit via internal rule
  Dot Product2 : DotProduct  OutDataTypeStr=Inherit: Inherit via internal rule
  Dot Product3 : DotProduct  OutDataTypeStr=Inherit: Inherit via internal rule
  Earth Radius : Constant  Value=ext_ENV_Re  VectorParams1D=off  SampleTime=0
  Gain : Gain  Gain=-1
  In Sun View : RelationalOperator  Operator=>  OutDataTypeStr=boolean  ZeroCross=off  RndMeth=Simplest  InputSameDT=off
  Max : MinMax  Function=max  Inputs=2
  Max1 : MinMax  Function=max  Inputs=2
  Sqrt1 : Sqrt
  Sqrt2 : Sqrt
  inView : Outport  SampleTime=0
  wires:
  Gain/1 -> Dot Product1/2, Divide/2, Dot Product1/1
  X_icrf/1 -> Divide2/2, Dot Product2/2, Dot Product2/1
  Earth Radius/1 -> Divide1/1
  Dot Product2/1 -> Sqrt1/1
  x_sun_icrf/1 -> Gain/1
  Max/1 -> Divide1/2, Divide2/1
  Divide1/1 -> Acos/1
  Acos/1 -> Acos1/1  "rho"
  Divide/1 -> Dot Product3/2
  Acos1/1 -> In Sun View/1
  Divide2/1 -> Dot Product3/1
  Dot Product3/1 -> In Sun View/2
  Dot Product1/1 -> Sqrt2/1
  Constant/1 -> Max/2
  In Sun View/1 -> inView/1
  Sqrt1/1 -> Max/1
  Sqrt2/1 -> Max1/1
  Max1/1 -> Divide/1
  Constant1/1 -> Max1/2

== system HSat_orbit_merged_maria/Subsystem1/Navigation/q_slo/VecNormalize ==
  In1 : Inport
  Constant : Constant
  Demux : Demux  Outputs=[-1 1]
  Divide : Product  Inputs=*/  OutDataTypeStr=double
  Ground : Ground
  Math Function : Math  Operator=square  SignedPower=on
  Math Function1 : Math  Operator=sqrt  SignedPower=on
  Mux : Mux  Inputs=2
  Mux1 : Mux  Inputs=2
  Product : Product  RndMeth=Zero
  Sum of Elements : Sum  Inputs=+
  Switch : Switch  Criteria=u2 > Threshold  Threshold=eps  SaturateOnIntegerOverflow=off  InputSameDT=off
  Out1 : Outport  VectorParamsAs1DForOutWhenUnconnected=off
  wires:
  Math Function/1 -> Sum of Elements/1
  Demux/1 -> Divide/1
  Constant/1 -> Mux1/2
  Mux1/1 -> Switch/3
  Divide/1 -> Out1/1
  Switch/1 -> Demux/1
  Mux/1 -> Switch/1
  Demux/2 -> Divide/2
  Product/1 -> Mux1/1
  In1/1 -> Product/1, Math Function/1, Mux/1
  Ground/1 -> Product/2
  Sum of Elements/1 -> Math Function1/1
  Math Function1/1 -> Mux/2, Switch/2

== system HSat_orbit_merged_maria/Subsystem1/Navigation/q_slo/VecNormalize1 ==
  In1 : Inport
  Constant : Constant
  Demux : Demux  Outputs=[-1 1]
  Divide : Product  Inputs=*/  OutDataTypeStr=double
  Ground : Ground
  Math Function : Math  Operator=square  SignedPower=on
  Math Function1 : Math  Operator=sqrt  SignedPower=on
  Mux : Mux  Inputs=2
  Mux1 : Mux  Inputs=2
  Product : Product  RndMeth=Zero
  Sum of Elements : Sum  Inputs=+
  Switch : Switch  Criteria=u2 > Threshold  Threshold=eps  SaturateOnIntegerOverflow=off  InputSameDT=off
  Out1 : Outport  VectorParamsAs1DForOutWhenUnconnected=off
  wires:
  Math Function/1 -> Sum of Elements/1
  Demux/1 -> Divide/1
  Constant/1 -> Mux1/2
  Mux1/1 -> Switch/3
  Divide/1 -> Out1/1
  Switch/1 -> Demux/1
  Mux/1 -> Switch/1
  Demux/2 -> Divide/2
  Product/1 -> Mux1/1
  In1/1 -> Product/1, Math Function/1, Mux/1
  Ground/1 -> Product/2
  Sum of Elements/1 -> Math Function1/1
  Math Function1/1 -> Mux/2, Switch/2

== system HSat_orbit_merged_maria/Subsystem1/Navigation/q_slo/VecNormalize2 ==
  In1 : Inport
  Constant : Constant
  Demux : Demux  Outputs=[-1 1]
  Divide : Product  Inputs=*/  OutDataTypeStr=double
  Ground : Ground
  Math Function : Math  Operator=square  SignedPower=on
  Math Function1 : Math  Operator=sqrt  SignedPower=on
  Mux : Mux  Inputs=2
  Mux1 : Mux  Inputs=2
  Product : Product  RndMeth=Zero
  Sum of Elements : Sum  Inputs=+
  Switch : Switch  Criteria=u2 > Threshold  Threshold=eps  SaturateOnIntegerOverflow=off  InputSameDT=off
  Out1 : Outport  VectorParamsAs1DForOutWhenUnconnected=off
  wires:
  Math Function/1 -> Sum of Elements/1
  Demux/1 -> Divide/1
  Constant/1 -> Mux1/2
  Mux1/1 -> Switch/3
  Divide/1 -> Out1/1
  Switch/1 -> Demux/1
  Mux/1 -> Switch/1
  Demux/2 -> Divide/2
  Product/1 -> Mux1/1
  In1/1 -> Product/1, Math Function/1, Mux/1
  Ground/1 -> Product/2
  Sum of Elements/1 -> Math Function1/1
  Math Function1/1 -> Mux/2, Switch/2

== system HSat_orbit_merged_maria/Subsystem1/Navigation/q_slo/VecNormalize3 ==
  In1 : Inport
  Constant : Constant
  Demux : Demux  Outputs=[-1 1]
  Divide : Product  Inputs=*/  OutDataTypeStr=double
  Ground : Ground
  Math Function : Math  Operator=square  SignedPower=on
  Math Function1 : Math  Operator=sqrt  SignedPower=on
  Mux : Mux  Inputs=2
  Mux1 : Mux  Inputs=2
  Product : Product  RndMeth=Zero
  Sum of Elements : Sum  Inputs=+
  Switch : Switch  Criteria=u2 > Threshold  Threshold=eps  SaturateOnIntegerOverflow=off  InputSameDT=off
  Out1 : Outport  VectorParamsAs1DForOutWhenUnconnected=off
  wires:
  Math Function/1 -> Sum of Elements/1
  Demux/1 -> Divide/1
  Constant/1 -> Mux1/2
  Mux1/1 -> Switch/3
  Divide/1 -> Out1/1
  Switch/1 -> Demux/1
  Mux/1 -> Switch/1
  Demux/2 -> Divide/2
  Product/1 -> Mux1/1
  In1/1 -> Product/1, Math Function/1, Mux/1
  Ground/1 -> Product/2
  Sum of Elements/1 -> Math Function1/1
  Math Function1/1 -> Mux/2, Switch/2

== system HSat_orbit_merged_maria/Subsystem1/Navigation/q_slo/Z x R ==
  a(1) a(2) a(3) : Inport
  b(1) b(2) b(3) : Inport  Port=2
  Product : Product  InputSameDT=on  SaturateOnIntegerOverflow=on  OutDataTypeStr=Inherit: Same as first input
  Product1 : Product  InputSameDT=on  SaturateOnIntegerOverflow=on  OutDataTypeStr=Inherit: Same as first input
  Selector : Selector  InputPortWidth=3  IndexOptions=Index vector (dialog)  Indices=[2 3 1]  OutputSizes=1
  Selector1 : Selector  InputPortWidth=3  IndexOptions=Index vector (dialog)  Indices=[3 1 2]  OutputSizes=1
  Selector2 : Selector  InputPortWidth=3  IndexOptions=Index vector (dialog)  Indices=[2 3 1]  OutputSizes=1
  Selector3 : Selector  InputPortWidth=3  IndexOptions=Index vector (dialog)  Indices=[3 1 2]  OutputSizes=1
  Sum : Sum  Inputs=+|-  InputSameDT=on  SaturateOnIntegerOverflow=on  OutDataTypeStr=Inherit: Same as first input
  c(1) c(2) c(3) : Outport  InitialOutput=0
  wires:
  Selector3/1 -> Product1/1
  Selector2/1 -> Product1/2
  Product1/1 -> Sum/2
  Selector1/1 -> Product/2
  Product/1 -> Sum/1
  a(1) a(2) a(3)/1 -> Selector3/1, Selector/1
  Selector/1 -> Product/1
  b(1) b(2) b(3)/1 -> Selector2/1, Selector1/1
  Sum/1 -> c(1) c(2) c(3)/1

== system HSat_orbit_merged_maria/Subsystem1/Navigation/q_slo/Z x Y ==
  a(1) a(2) a(3) : Inport
  b(1) b(2) b(3) : Inport  Port=2
  Product : Product  InputSameDT=on  SaturateOnIntegerOverflow=on  OutDataTypeStr=Inherit: Same as first input
  Product1 : Product  InputSameDT=on  SaturateOnIntegerOverflow=on  OutDataTypeStr=Inherit: Same as first input
  Selector : Selector  InputPortWidth=3  IndexOptions=Index vector (dialog)  Indices=[2 3 1]  OutputSizes=1
  Selector1 : Selector  InputPortWidth=3  IndexOptions=Index vector (dialog)  Indices=[3 1 2]  OutputSizes=1
  Selector2 : Selector  InputPortWidth=3  IndexOptions=Index vector (dialog)  Indices=[2 3 1]  OutputSizes=1
  Selector3 : Selector  InputPortWidth=3  IndexOptions=Index vector (dialog)  Indices=[3 1 2]  OutputSizes=1
  Sum : Sum  Inputs=+|-  InputSameDT=on  SaturateOnIntegerOverflow=on  OutDataTypeStr=Inherit: Same as first input
  c(1) c(2) c(3) : Outport  InitialOutput=0
  wires:
  Selector3/1 -> Product1/1
  Selector2/1 -> Product1/2
  Product1/1 -> Sum/2
  Selector1/1 -> Product/2
  Product/1 -> Sum/1
  a(1) a(2) a(3)/1 -> Selector3/1, Selector/1
  Selector/1 -> Product/1
  b(1) b(2) b(3)/1 -> Selector2/1, Selector1/1
  Sum/1 -> c(1) c(2) c(3)/1

== system HSat_orbit_merged_maria/Subsystem1/control/EORattitude/OR or SK unloading ==
  AmomECI : Inport
  SKunload : Inport  Port=2
  Compare To Constant : simulink/Logic and Bit Operations/Compare To Constant  relop=>  const=0.1  OutDataTypeStr=boolean
  Dot Product : DotProduct  OutDataTypeStr=Inherit: Inherit via internal rule
  Logical Operator : Logic  AllPortsSameDT=off  OutDataTypeStr=boolean
  NOT : Logic  Operator=NOT  IconShape=distinctive  AllPortsSameDT=off  OutDataTypeStr=boolean
  Scope : Scope
  Sqrt : Sqrt
  PPU1active : Outport
  PPU2active : Outport  Port=2
  PPUSKactive : Outport  Port=3
  wires:
  SKunload/1 -> NOT/1, Logical Operator/1
  NOT/1 -> PPU1active/1, PPU2active/1
  AmomECI/1 -> Dot Product/2, Dot Product/1
  Sqrt/1 -> Scope/1, Compare To Constant/1
  Dot Product/1 -> Sqrt/1
  Compare To Constant/1 -> Logical Operator/2
  Logical Operator/1 -> PPUSKactive/1

== system HSat_orbit_merged_maria/Subsystem1/control/EORattitude/Subsystem ==
  AmomECI : Inport
  q_eci2scb : Inport  Port=2
  EORthrustSCB : Inport  Port=3
  EORtorqueSCB : Inport  Port=4
  thrust_slo : Inport  Port=5
  q_slo2eci : Inport  Port=6
  sunv_eci : Inport  Port=7
  Quaternion Rotation1 : aerolibutil/Quaternion Rotation
  Subsystem1 : Subsystem
  Subsystem3 : Subsystem
  qECI2scb : Outport
  DoAMOM : Outport  Port=2
  NoAMOM : Outport  Port=3
  wires:
  q_slo2eci/1 -> Subsystem1/4(q_slo2eci)
  EORthrustSCB/1 -> Subsystem1/2(EORthrustSCB)
  sunv_eci/1 -> Subsystem1/5(sunv_eci)
  EORtorqueSCB/1 -> Subsystem3/2(EORtorqueSCB)
  thrust_slo/1 -> Subsystem1/3(thrust_slo)
  AmomECI/1 -> Quaternion Rotation1/2
  Subsystem1/1(qECI2scb) -> qECI2scb/1
  Subsystem3/3(FlipPlusMinus) -> Subsystem1/1(Flipsign)
  Quaternion Rotation1/1 -> Subsystem3/1(AmomSCB)  "amomscb"
  q_eci2scb/1 -> Quaternion Rotation1/1
  Subsystem3/1(DoAMOM) -> DoAMOM/1
  Subsystem3/2(NoAMOM) -> NoAMOM/1

== system HSat_orbit_merged_maria/Subsystem1/control/EORattitude/Subsystem2 ==
  note: Thrust and torque due to
      | thrusters
  PPU1active : Inport
  AllThrustsSCB : Inport  Port=2
  PPU2active : Inport  Port=3
  AllTorquesSCB1 : Inport  Port=4
  PPUSKactive : Inport  Port=5
  Constant1 : Constant  Value=3
  Constant2 : Constant  Value=3
  Constant7 : Constant
  Logical Operator : Logic  AllPortsSameDT=off  OutDataTypeStr=boolean
  Logical Operator1 : Logic  AllPortsSameDT=off  OutDataTypeStr=boolean
  Logical Operator2 : Logic  Operator=OR  Inputs=3  AllPortsSameDT=off  OutDataTypeStr=boolean
  Logical Operator3 : Logic  AllPortsSameDT=off  OutDataTypeStr=boolean
  PPU1 : Subsystem
  PPU3 : Subsystem
  PPU_SK : Subsystem
  Product{,1..5} (6 alike) : Product
  Sum1 : Sum  Inputs=+++
  Sum2 : Sum  Inputs=+++
  thurst and torque for 3 SK thrusters : Subsystem
  thurst and torque for each OR thruster : Subsystem
  ActiveThrusters : Outport
  EORForceSCB : Outport  Port=2
  EORTorqueSCB : Outport  Port=3
  SKThrustersActive : Outport  Port=4
  wires:
  AllTorquesSCB1/1 -> thurst and torque for 3 SK thrusters/2(AllTorquesSCB), thurst and torque for each OR thruster/2(AllTorquesSCB)
  Sum1/1 -> EORForceSCB/1
  Product2/1 -> Sum2/1
  PPU3/2(TorqueSCB) -> Product3/2
  PPU3/1(ForceSCB) -> Product1/2
  Sum2/1 -> EORTorqueSCB/1
  PPU1/1(ForceSCB) -> Product/2
  thurst and torque for each OR thruster/2(TorquesORSCB) -> PPU3/3(TorqueORSCB), PPU1/3(TorqueORSCB)
  PPU1/2(TorqueSCB) -> Product2/2
  Constant1/1 -> PPU3/2(OR ThrustNo)
  Logical Operator2/1 -> ActiveThrusters/1
  thurst and torque for each OR thruster/1(ForceORSCB) -> PPU3/1(ForceORSCB), PPU1/1(ForceORSCB)
  PPU3/3(activethrusters) -> Logical Operator1/2
  AllThrustsSCB/1 -> thurst and torque for 3 SK thrusters/1(AllForcesSCB), thurst and torque for each OR thruster/1(AllForcesSCB)
  Logical Operator/1 -> Logical Operator2/1
  PPU2active/1 -> Product3/1, Logical Operator1/1, Product1/1
  Product1/1 -> Sum1/2
  Logical Operator1/1 -> Logical Operator2/3
  Product/1 -> Sum1/1
  PPU1/3(activethrusters) -> Logical Operator/2
  PPU1active/1 -> Product2/1, Logical Operator/1, Product/1
  Constant7/1 -> PPU1/2(OR ThrustNo)
  Product3/1 -> Sum2/2
  thurst and torque for 3 SK thrusters/2(TorquesSKSCB) -> PPU_SK/3(TorqueSKSCB)
  thurst and torque for 3 SK thrusters/1(ForceSKSCB) -> PPU_SK/1(ForceSKSCB)
  Constant2/1 -> PPU_SK/2(SK ThrustNo)
  PPU_SK/1(ForceSCB) -> Product4/1
  PPUSKactive/1 -> Logical Operator3/2, Product4/2, Product5/2
  Product4/1 -> Sum1/3
  PPU_SK/2(TorqueSCB) -> Product5/1
  Product5/1 -> Sum2/3
  PPU_SK/3(activethrusters) -> Logical Operator3/1, SKThrustersActive/1
  Logical Operator3/1 -> Logical Operator2/2

== system HSat_orbit_merged_maria/Subsystem1/control/EORattitude/Subsystem4 ==
  AmomECI : Inport
  EORthrustSCB : Inport  Port=2
  EORtorqueSCB : Inport  Port=3
  thrust_slo : Inport  Port=4
  q_eci2slo : Inport  Port=5
  sunv_eci : Inport  Port=6
  unloading_ongoing : Inport  Port=7
  Attitude for OR thrusters : Subsystem
  Attitude for SK unloading : Subsystem
  Bus Creator : BusCreator  Inputs=4
  Constant : Constant
  Constant1 : Constant  Value=0
  Display : Display
  Quaternion Multiplication2 : aerolibutil/Quaternion Multiplication
  Quaternion Rotation1 : aerolibutil/Quaternion Rotation
  Scope : Scope
  Subsystem3 : Subsystem
  Switch : Switch  Criteria=u2 > Threshold  SaturateOnIntegerOverflow=off  InputSameDT=off
  Switch1 : Switch  Criteria=u2 > Threshold  SaturateOnIntegerOverflow=off  InputSameDT=off
  Switch2 : Switch  Criteria=u2 > Threshold  SaturateOnIntegerOverflow=off  InputSameDT=off
  Unit Delay : UnitDelay  SampleTime=-1  HasFrameUpgradeWarning=on
  Unit Delay1 : UnitDelay  SampleTime=-1  HasFrameUpgradeWarning=on
  flips around thrust vector : Subsystem
  "use q from thrust calc " : Subsystem
  qECI2scb : Outport
  DoAMOM : Outport  Port=2
  NoAMOM : Outport  Port=3
  flip_unloading : Outport  Port=4
  SKunload : Outport  Port=5
  wires:
  AmomECI/1 -> Subsystem3/2(AmomECI), Attitude for SK unloading/2(AmomECI), Quaternion Rotation1/2
  Quaternion Rotation1/1 -> Subsystem3/3(AmomSCB)  "amomscb"
  EORthrustSCB/1 -> Attitude for OR thrusters/4(thrustscb), Subsystem3/1(thrustscb), flips around thrust vector/1(thrustscb)  "thrustscb"
  EORtorqueSCB/1 -> Attitude for SK unloading/1(SKtorqueSCB), Subsystem3/4(EORtorqueSCB)
  Subsystem3/1(Flipyaxis) -> Switch1/2  "flip"
  flips around thrust vector/1(qflipscb) -> Switch1/1
  "use q from thrust calc "/1(qflipscb) -> Switch1/3
  Switch1/1 -> Quaternion Multiplication2/2
  Quaternion Multiplication2/1 -> Switch/3
  Unit Delay1/1 -> Quaternion Rotation1/1
  Attitude for OR thrusters/1(q*r) -> Quaternion Multiplication2/1
  q_eci2slo/1 -> Attitude for OR thrusters/1(q_eci2slo)
  thrust_slo/1 -> Attitude for OR thrusters/2(thrust_vec_slo)
  sunv_eci/1 -> Attitude for SK unloading/3(sunv_eci), Attitude for OR thrusters/3(sunvECI)
  Subsystem3/2(DoAMOM) -> DoAMOM/1
  Subsystem3/3(NoAMOM) -> NoAMOM/1
  Subsystem3/4(worstRwMom) -> Bus Creator/3  "worstRwMom"
  Subsystem3/5(SKunload) -> Unit Delay/1, SKunload/1, Bus Creator/2, Switch2/2  "SKunloading"
  Unit Delay/1 -> Switch/2
  Attitude for SK unloading/1(q_ECI2scb) -> Switch/1
  Switch/1 -> Unit Delay1/1, qECI2scb/1
  unloading_ongoing/1 -> Subsystem3/5(unloading_ongoing)
  Constant/1 -> Switch2/1
  Constant1/1 -> Switch2/3
  Switch2/1 -> Scope/1, Display/1
  Subsystem3/6(idxMinMom) -> Bus Creator/4  "idxMinMom"
  Bus Creator/1 -> flip_unloading/1
  Subsystem3/7(flip_now) -> Bus Creator/1  "flip"

== system HSat_orbit_merged_maria/Subsystem1/control/Subsystem6/Subsystem2 ==
  PPU1active : Inport
  PPU2active : Inport  Port=2
  AllTorquesSCB : Inport  Port=3
  q_eci2scb_wanted : Inport  Port=4
  WantedTorqueECI : Inport  Port=5
  sunv : Inport  Port=6
  Multiport Switch : MultiPortSwitch  SaturateOnIntegerOverflow=off  InputSameDT=off
  Multiport Switch1 : MultiPortSwitch  SaturateOnIntegerOverflow=off  InputSameDT=off
  PPU1 : Subsystem
  PPU1+2 : Subsystem
  PPU2 : Subsystem
  Subsystem : Subsystem
  Subsystem1 : Subsystem
  Sum1 : Sum  Inputs=++|
  ActiveThrusters : Outport
  q_eci2scb : Outport  Port=2
  wires:
  Multiport Switch1/1 -> ActiveThrusters/1
  PPU1active/1 -> Sum1/1
  PPU2active/1 -> Sum1/2
  PPU1+2/2(activethrusters) -> Multiport Switch1/4
  PPU1/2(activethrusters) -> Multiport Switch1/2
  PPU1/1(torqueSCB) -> Multiport Switch/2  "torquescb"
  PPU1+2/1(torqueSCB) -> Multiport Switch/4  "torquescb"
  PPU2/2(activethrusters) -> Multiport Switch1/3
  Sum1/1 -> Multiport Switch/1, Multiport Switch1/1
  WantedTorqueECI/1 -> Subsystem1/2(WantedTorqueECI), PPU1+2/2(WantedTorqueECI), PPU2/2(WantedTorqueECI), PPU1/2(WantedTorqueECI)
  PPU2/1(torqueSCB) -> Multiport Switch/3  "torquescb"
  Subsystem/1(TorqueSKECI) -> PPU1+2/1(TorqueSKECI), PPU2/1(TorqueSKECI), PPU1/1(TorqueSKECI)
  q_eci2scb_wanted/1 -> Subsystem/2(q_eci2scb_wanted)
  AllTorquesSCB/1 -> Subsystem/1(AllTorquesSCB)
  Subsystem1/1(q_eci2scb) -> q_eci2scb/1
  sunv/1 -> Subsystem1/3(sunvECI)
  Multiport Switch/1 -> Subsystem1/1(TorqueSCB)

== system HSat_orbit_merged_maria/Subsystem1/control/TorquesAndForces/Subsystem ==
  SC_mass : Inport
  Constant1 : Constant  Value=sim_SC_init_CoG_EOR_dry
  Constant2 : Constant  Value=sim_SC_init_CoG_propellant
  Constant3 : Constant  Value=sim_SC_init_dry_mass
  Constant4 : Constant  Value=sim_SC_init_dry_mass
  Divide : Product  Inputs=/*
  Product : Product
  Product1 : Product
  Reshape : Reshape  OutputDimensionality=Row vector (2-D)
  Sum : Sum  Inputs=+-|
  Sum1 : Sum  Inputs=+|+
  SC_CoG : Outport
  wires:
  Constant4/1 -> Sum/2
  Product1/1 -> Sum1/2
  Constant3/1 -> Product1/1
  SC_mass/1 -> Divide/1, Sum/1
  Constant1/1 -> Product1/2
  Product/1 -> Sum1/1
  Sum1/1 -> Divide/2
  Constant2/1 -> Product/2
  Sum/1 -> Product/1  "propellant mass"
  Divide/1 -> Reshape/1
  Reshape/1 -> SC_CoG/1

== system HSat_orbit_merged_maria/Subsystem1/Dynamics/Subsystem/3 body perturbation legendre polynomial/Subsystem1 ==
  sat : Inport
  3 body : Inport  Port=2
  mass : Inport  Port=3
  Legendre deg : Inport  Port=4
  Constant : Constant  Value=6.6743e-11
  Divide : Product  Inputs=/*
  Divide1 : Product  Inputs=*/
  Dot Product : DotProduct  OutDataTypeStr=Inherit: Inherit via internal rule
  Dot Product1 : DotProduct  OutDataTypeStr=Inherit: Inherit via internal rule
  Dot Product2 : DotProduct  OutDataTypeStr=Inherit: Inherit via internal rule
  MATLAB Function : MATLAB Function  TreatAsAtomicUnit=on
  Product{,1..3} (4 alike) : Product
  Sqrt : Sqrt
  Sqrt1 : Sqrt
  Subtract : Sum  Inputs=-+
  Subtract1 : Sum  Inputs=+-
  cos angle : Subsystem
  Out1 : Outport
  wires:
  sat/1 -> cos angle/1(sat), Subtract/2, Subtract1/2, Dot Product2/2, Dot Product2/1  "r_sat"
  3 body/1 -> Dot Product1/1, Dot Product/2, Dot Product/1, Dot Product1/2, Subtract1/1, cos angle/2(3 body)  "r_3body"
  cos angle/1(cos angle) -> MATLAB Function/1(costheta)
  Legendre deg/1 -> MATLAB Function/2(degree)
  Divide/1 -> MATLAB Function/3(h)
  mass/1 -> Product/2
  Constant/1 -> Product/1
  Product/1 -> Divide1/1  "mu_3body"
  Divide1/1 -> Product1/1
  Product1/1 -> Out1/1
  MATLAB Function/1(beta) -> Product2/1
  Subtract1/1 -> Product2/2  "r_sat3body"
  Product2/1 -> Subtract/1
  Subtract/1 -> Product1/2
  Dot Product/1 -> Product3/1
  Product3/1 -> Divide1/2
  Dot Product1/1 -> Sqrt/1
  Sqrt/1 -> Divide/1, Product3/2  "| r_3body |"
  Dot Product2/1 -> Sqrt1/1
  Sqrt1/1 -> Divide/2  "| r_sat |"

== system HSat_orbit_merged_maria/Subsystem1/Dynamics/Subsystem/3 body perturbation legendre polynomial/Subsystem2 ==
  sat : Inport
  3 body : Inport  Port=2
  mass : Inport  Port=3
  Legendre deg : Inport  Port=4
  Constant : Constant  Value=ext_ENV_G
  Divide : Product  Inputs=/*
  Divide1 : Product  Inputs=*/
  Dot Product : DotProduct  OutDataTypeStr=Inherit: Inherit via internal rule
  Dot Product1 : DotProduct  OutDataTypeStr=Inherit: Inherit via internal rule
  Dot Product2 : DotProduct  OutDataTypeStr=Inherit: Inherit via internal rule
  MATLAB Function : MATLAB Function  TreatAsAtomicUnit=on
  Product{,1..3} (4 alike) : Product
  Sqrt : Sqrt
  Sqrt1 : Sqrt
  Subtract : Sum  Inputs=-+
  Subtract1 : Sum  Inputs=+-
  cos angle : Subsystem
  Out1 : Outport
  wires:
  sat/1 -> cos angle/1(sat), Subtract/2, Subtract1/2, Dot Product2/2, Dot Product2/1  "r_sat"
  3 body/1 -> Dot Product1/1, Dot Product/2, Dot Product/1, Dot Product1/2, Subtract1/1, cos angle/2(3 body)  "r_3body"
  cos angle/1(cos angle) -> MATLAB Function/1(costheta)
  Legendre deg/1 -> MATLAB Function/2(degree)
  Divide/1 -> MATLAB Function/3(h)
  mass/1 -> Product/2
  Constant/1 -> Product/1
  Product/1 -> Divide1/1  "mu_3body"
  Divide1/1 -> Product1/1
  Product1/1 -> Out1/1
  MATLAB Function/1(beta) -> Product2/1
  Subtract1/1 -> Product2/2  "r_sat3body"
  Product2/1 -> Subtract/1
  Subtract/1 -> Product1/2
  Dot Product/1 -> Product3/1
  Product3/1 -> Divide1/2
  Dot Product1/1 -> Sqrt/1
  Sqrt/1 -> Divide/1, Product3/2  "| r_3body |"
  Dot Product2/1 -> Sqrt1/1
  Sqrt1/1 -> Divide/2  "| r_sat |"
